simulink model "multiplexer_circuit"  (R2020a)
settings: Solver=VariableStepAuto  StartTime=0.0  StopTime=inf  RelTol=1e-3
settings Model: Creator=F1  LastModifiedBy=F1

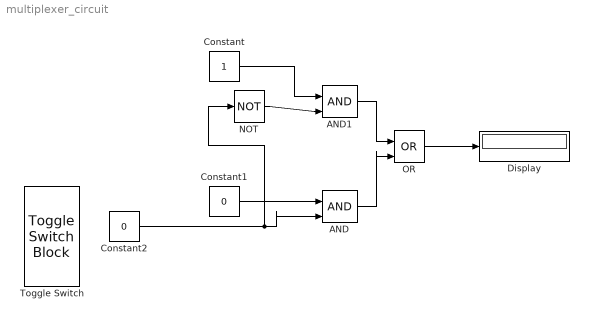
== system multiplexer_circuit ==
  AND : Logic  IconShape=distinctive  AllPortsSameDT=off  OutDataTypeStr=boolean
  AND1 : Logic  IconShape=distinctive  AllPortsSameDT=off  OutDataTypeStr=boolean
  Constant : Constant
  Constant1 : Constant  Value=0
  Constant2 : Constant  Value=0
  Display : Display
  NOT : Logic  Operator=NOT  IconShape=distinctive  AllPortsSameDT=off  OutDataTypeStr=boolean
  OR : Logic  Operator=OR  IconShape=distinctive  AllPortsSameDT=off  OutDataTypeStr=boolean
  Toggle Switch : ToggleSwitchBlock
      settings: Values={{'Off', 'On'}, [0 1]}
  wires:
  Constant2/1 -> NOT/1, AND/2
  Constant1/1 -> AND/1
  NOT/1 -> AND1/2
  Constant/1 -> AND1/1
  AND1/1 -> OR/1
  AND/1 -> OR/2
  OR/1 -> Display/1
